simulink library "mss_wrappers"  (R2024a)
settings: Solver=VariableStepAuto  StartTime=0.0  StopTime=10.0  RelTol=1e-3
settings Model: Creator=luka  LastModifiedBy=luka

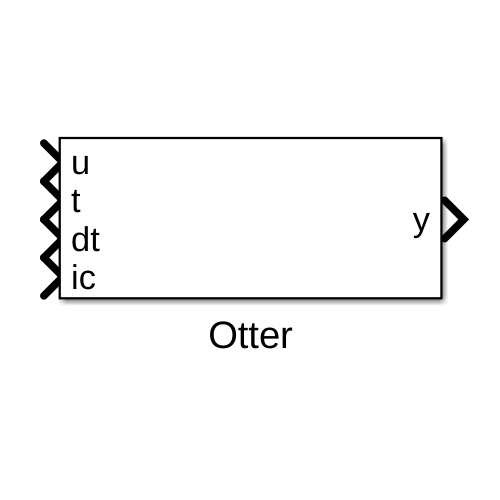
[thumbnail: Simulink's stored preview of the top-level diagram]
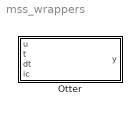
== system mss_wrappers ==
  Otter : Subsystem  Tag=system;__cs_slx_sys;  mask{payload_mass=0, payload_location=[0,0, 0], current_speed=0, current_direction=0, out_gain=1}
      mask prompts: payload_mass "Payload mass"; payload_location "Payload location"; current_speed "Current speed"; current_direction "Current direction"

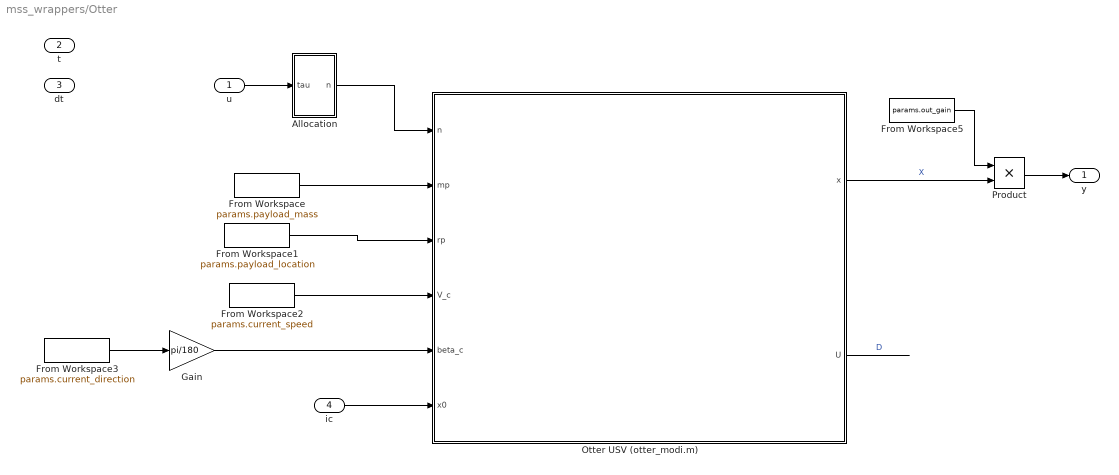
== system mss_wrappers/Otter ==
  u : Inport  PortDimensions=2
  t : Inport  Port=2
  dt : Inport  Port=3
  ic : Inport  Port=4
  Allocation : Subsystem
  From Workspace : FromWorkspace  VariableName=params.payload_mass  SampleTime=-1  OutputAfterFinalValue=Holding final value
  From Workspace1 : FromWorkspace  VariableName=params.payload_location  SampleTime=-1  OutputAfterFinalValue=Holding final value
  From Workspace2 : FromWorkspace  VariableName=params.current_speed  SampleTime=-1  OutputAfterFinalValue=Holding final value
  From Workspace3 : FromWorkspace  VariableName=params.current_direction  SampleTime=-1  OutputAfterFinalValue=Holding final value
  From Workspace5 : FromWorkspace  VariableName=params.out_gain  SampleTime=-1  OutputAfterFinalValue=Holding final value
  Gain : Gain  Gain=pi/180
  "Otter USV (otter_modi.m) " : Subsystem  AncestorBlock=mssSimulink/Marine craft models/Otter USV (otter.m)
      settings: LibrarySourceBlock=mssSimulink/Marine craft models/Otter USV (otter.m)
      mask Display: image('otter.jpg'); % Use "Edit Image" on toolstrip to change.
  Product : Product
  y : Outport  PortDimensions=12
  wires:
  From Workspace3/1 -> Gain/1
  "Otter USV (otter_modi.m) "/2(U) -> ?  "D"
  Allocation/1(n) -> "Otter USV (otter_modi.m) "/1(n)
  From Workspace2/1 -> "Otter USV (otter_modi.m) "/4(V_c)
  "Otter USV (otter_modi.m) "/1(x) -> Product/2  "X"
  ic/1 -> "Otter USV (otter_modi.m) "/6(x0)
  From Workspace1/1 -> "Otter USV (otter_modi.m) "/3(rp)
  Gain/1 -> "Otter USV (otter_modi.m) "/5(beta_c)
  u/1 -> Allocation/1(tau)
  From Workspace/1 -> "Otter USV (otter_modi.m) "/2(mp)
  Product/1 -> y/1
  From Workspace5/1 -> Product/1

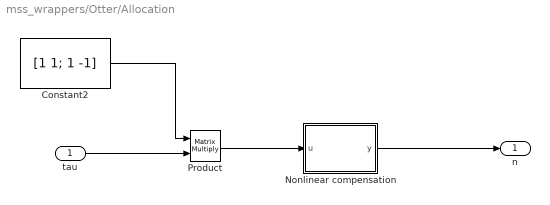
== system mss_wrappers/Otter/Allocation ==
  tau : Inport
  Constant2 : Constant  Value=[1 1; 1 -1]
  Nonlinear compensation : MATLAB Function  TreatAsAtomicUnit=on
  Product : Product  Multiplication=Matrix(*)
  n : Outport
  wires:
  Constant2/1 -> Product/1
  Nonlinear compensation/1(y) -> n/1
  tau/1 -> Product/2
  Product/1 -> Nonlinear compensation/1(u)

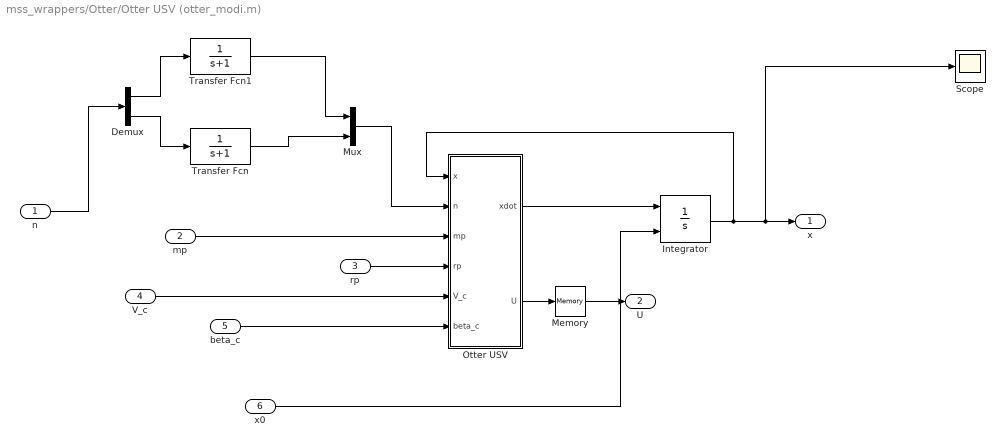
== system mss_wrappers/Otter/Otter USV (otter_modi.m)  ==
  n : Inport
  mp : Inport  Port=2
  rp : Inport  Port=3
  V_c : Inport  Port=4
  beta_c : Inport  Port=5
  x0 : Inport  Port=6
  Demux : Demux  Outputs=2
  Integrator : Integrator  InitialConditionSource=external  InitialCondition=[1 1]  UpperSaturationLimit=10  LowerSaturationLimit=-10
  Memory : Memory
  Mux : Mux  Inputs=2
  Otter USV : MATLAB Function  TreatAsAtomicUnit=on
  Scope : Scope
  Transfer Fcn : TransferFcn  Denominator=[1 1]
  Transfer Fcn1 : TransferFcn  Denominator=[1 1]
  x : Outport
  U : Outport  Port=2
  wires:
  Transfer Fcn1/1 -> Mux/1
  Transfer Fcn/1 -> Mux/2
  Demux/2 -> Transfer Fcn/1
  Demux/1 -> Transfer Fcn1/1
  V_c/1 -> Otter USV/5(V_c)
  Otter USV/2(U) -> Memory/1
  mp/1 -> Otter USV/3(mp)
  Otter USV/1(xdot) -> Integrator/1
  beta_c/1 -> Otter USV/6(beta_c)
  rp/1 -> Otter USV/4(rp)
  x0/1 -> Integrator/2
  Memory/1 -> U/1
  n/1 -> Demux/1
  Mux/1 -> Otter USV/2(n)
  Integrator/1 -> Otter USV/1(x), Scope/1, x/1

== matlab function mss_wrappers/Otter/Allocation/Nonlinear compensation ==
  data: u input; y output
function y = fcn(u)

gain_pos = 1.0802e+04;
gain_neg = -1.0350e+04;
y = zeros(2, 1);
for i=1:2
    if u(i) > 0
        y(i) = sqrt(gain_pos * u(i));
    else
        y(i) = -sqrt(gain_neg * u(i));
    end
end
end

== matlab function mss_wrappers/Otter/Otter USV (otter_modi.m) /Otter USV ==
  settings: updateMethod=DISCRETE
  data: x input; n input; xdot output; mp input; rp input; V_c input; beta_c input; U output
function [xdot, U] = fcn(x,n,mp,rp,V_c,beta_c)

[xdot,U] = otter(x,n,mp,rp,V_c,beta_c);

end
